simulink model "digit"  (R2022b)
settings: Solver=ode1  StartTime=0.0  StopTime=inf  FixedStep=0.001  RelTol=1e-3
settings Model: Creator=user  LastModifiedBy=user

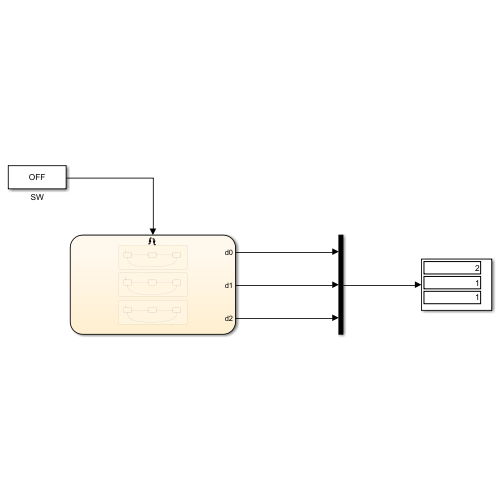
[thumbnail: Simulink's stored preview of the top-level diagram]
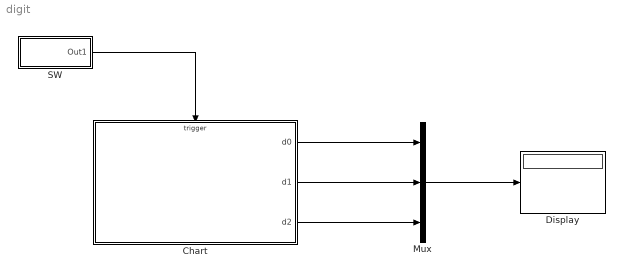
== system digit ==
  Chart : Stateflow chart  TreatAsAtomicUnit=on
  Display : Display
  Mux : Mux  Inputs=3
  SW : Subsystem  StartFcn=|  mask{str=OFF}
      | set_param(gcb, 'str', 'OFF');
      | set_param([gcb '/Constant'], 'Value', '0');
      mask prompts: str "Display name:"
      settings: OpenFcn=|
      | old_val = get_param([gcb '/Constant'], 'Value');
      | 
      | switch old_val
      | case '0'
      |     set_param(gcb, 'str', 'ON');
      |     set_param([gcb '/Constant'], 'Value', '1');
      | 
      | case '1'
      |     set_param(gcb, 'str', 'OFF');
      |     set_param([gcb '/Constant'], 'Value', '0');
      | 
      | otherwise
      |     set_param(gcb, 'str', 'ON');
      |     set_param([gcb '/Constant'], 'Value', '0');
      | 
      | end
      mask DialogControl ParameterGroupVar Prompt: 파라미터
      mask Display: disp(get_param(gcb,'str'));
  wires:
  SW/1(Out1) -> Chart/Trigger
  Chart/1(d0) -> Mux/1
  Chart/3(d2) -> Mux/3
  Chart/2(d1) -> Mux/2
  Mux/1 -> Display/1

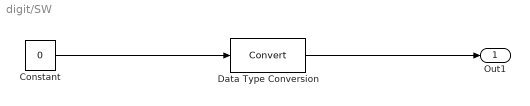
== system digit/SW ==
  Constant : Constant  Value=0
  Data Type Conversion : DataTypeConversion  SaturateOnIntegerOverflow=off  RndMeth=Floor
  Out1 : Outport
  wires:
  Data Type Conversion/1 -> Out1/1
  Constant/1 -> Data Type Conversion/1

== stateflow chart digit/Chart ==
  settings: executeAtInitialization=1
  state digit0 [parallel]
    settings: executionOrder=1
    state zero
      en:
      d0 = 0;
    state one
      en:
      d0 = 1;
    state two
      en:
      d0 = 2;
    (default) -> digit0.zero
    digit0.zero -> digit0.one : CLK
    digit0.one -> digit0.two : CLK
    digit0.two -> digit0.zero : CLK /{CLK_D1}
  state digit1 [parallel]
    settings: executionOrder=2
    state zero
      en:
      d1 = 0;
    state one
      en:
      d1 = 1;
    state two
      en:
      d1 = 2;
    (default) -> digit1.zero
    digit1.zero -> digit1.one : CLK_D1
    digit1.one -> digit1.two : CLK_D1
    digit1.two -> digit1.zero : CLK_D1 /{CLK_D2}
  state digit2 [parallel]
    settings: executionOrder=3
    state zero
      en:
      d2 = 0;
    state one
      en:
      d2 = 1;
    state two
      en:
      d2 = 2;
    (default) -> digit2.zero
    digit2.zero -> digit2.one : CLK_D2
    digit2.one -> digit2.two : CLK_D2
    digit2.two -> digit2.zero : CLK_D2
  data: d0 output; d1 output; d2 output
  events: CLK_D1 local FUNCTION_CALL_EVENT; CLK input EITHER_EDGE_EVENT; CLK_D2 local FUNCTION_CALL_EVENT
